simulink model "Avi_PWMSYN"  (Simulink 7.3)
settings: Solver=ode23tb  StartTime=0.0  StopTime=.25  RelTol=1e-3
libraries: powerlib x24, simulink x1
settings Model: Creator=ADMIN  LastModifiedBy=ADMIN

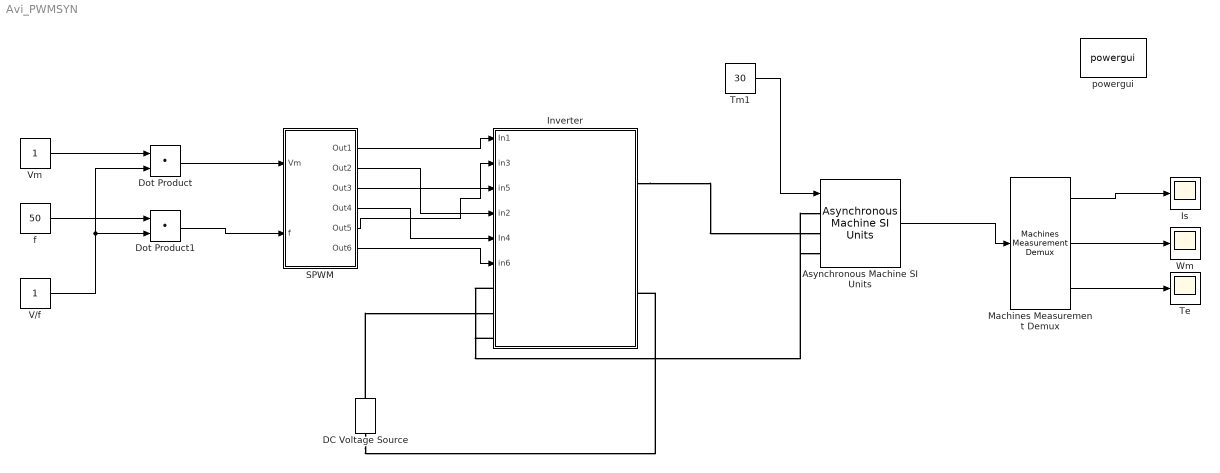
== system Avi_PWMSYN ==
  Asynchronous Machine SI Units : powerlib/Machines/Asynchronous Machine SI Units  DialogController=POWERSYS.PowerSysDialog  SystemSampleTime=-1  PresetModel=No  MechanicalLoad=Torque Tm  ShowDetailedParameters=on  RotorType=Squirrel-cage  ReferenceFrame=Stationary  NominalParameters=[ 3746 220 50 ]  Stator=[.453 2e-3]  Rotor=[ .816 2e-3]  Lm=.0631  Mechanical=[ .089 0 2 ]  PolePairs=2  InitialConditions=[1 0 0 0 0 0 0 0]  Units=SI  LoadFlowParameters=1492000  SimulateSaturation=off  Saturation=[14.03593122, 27.81365428, 53.79336849, 72.68890987, 97.98006896, 148.6815601, 215.7428561, 302.9841135, 428.7778367 ; 230, 322, 414, 460, 506, 552, 598, 644, 690]  TsPowergui=0  TsBlock=-1  IterativeModel=Forward Euler
  DC Voltage Source : powerlib/Electrical Sources/DC Voltage Source  DialogController=POWERSYS.PowerSysDialog  SystemSampleTime=-1  Amplitude=250  Measurements=None
  Dot Product : DotProduct  OutDataType=fixdt(1, 16)  OutScaling=2^-10  InputSameDT=on  OutDataTypeStr=Inherit: Inherit via internal rule
  Dot Product1 : DotProduct  OutDataType=fixdt(1, 16)  OutScaling=2^-10  InputSameDT=on  OutDataTypeStr=Inherit: Inherit via internal rule
  Inverter : Subsystem
  Is : Scope
      settings: YMin=-40  YMax=40  SaveName=ScopeData4
  Machines Measurement Demux : powerlib/Machines/Machines Measurement Demux  DialogController=POWERSYS.PowerSysDialog  SystemSampleTime=-1  machType=Asynchronous  ssm1=on  ssm2=on  ssm3=on  ssm4=on  ssm5=on  ssm6=on  sm1=on  sm2=off  sm3=off  sm4=off  sm5=off  sm6=off  sm7=off  sm8=on  sm9=off  sm10=off  sm11=off  sm115=on  sm12=off  sm13=off  sm14=off  asm1=off  asm2=off  asm3=off  asm4=off  asm5=on  asm6=off  asm7=off  asm8=off  asm9=on  asm10=on  asm11=off  pmsm1=on  pmsm2=on  pmsm3=on  pmsm4=off  pmsm5=on  pmsm6=on  pmsm7=on  lastType=1
  SPWM : Subsystem
  Te : Scope
      settings: YMin=10  YMax=100  SaveName=ScopeData6
  Tm1 : Constant  Value=30  OutDataType=fixdt(1, 16)  OutScaling=2^0
  V/f : Constant  OutDataType=fixdt(1, 16)  OutScaling=2^0
  Vm : Constant  OutDataType=fixdt(1, 16)  OutScaling=2^0
  Wm : Scope
      settings: YMin=0  YMax=20  SaveName=ScopeData5
  f : Constant  Value=50  OutDataType=fixdt(1, 16)  OutScaling=2^0
  powergui : powerlib/powergui  Priority=1  SystemSampleTime=-1  SimulationMode=Continuous  SampleTime=50e-6  frequency=60  SPID=off  DisableSnubberDevices=off  DisableRonSwitches=off  DisableVfSwitches=off  SwTol=0  Interpol=off  frequencyindice=0  echomessages=off  HookPort=off  DisplayEquations=off  FunctionMessages=off  EnableUseOfTLC=off  x0status=blocks  RestoreLinks=warning  Frange=[0:2:500]  Ylog=off  Xlog=on  ShowGrid=off  save=off  variable=ZData  ZoomFFT=on  StartTime=0.0  cycles=1  DisplayStyle=1  fundamental=60  FreqAxis=off  MaxFrequency=1000  frequencyindicesteady=1  RmsSteady=1  display=off  Ts=0  methode=off
  wires:
  Vm/1 -> Dot Product/1
  f/1 -> Dot Product1/1
  V/f/1 -> Dot Product1/2, Dot Product/2
  Dot Product/1 -> SPWM/1(Vm)
  Dot Product1/1 -> SPWM/2(f)
  SPWM/1(Out1) -> Inverter/1(In1)
  SPWM/2(Out2) -> Inverter/4(in2)
  SPWM/3(Out3) -> Inverter/2(in3)
  SPWM/4(Out4) -> Inverter/5(In4)
  SPWM/5(Out5) -> Inverter/3(in5)
  SPWM/6(Out6) -> Inverter/6(in6)
  Tm1/1 -> Asynchronous Machine SI Units/1
  Asynchronous Machine SI Units/1 -> Machines Measurement Demux/1
  Machines Measurement Demux/1 -> Is/1
  Machines Measurement Demux/2 -> Wm/1
  Machines Measurement Demux/3 -> Te/1
  connections:
  Inverter/LConn1 -- Asynchronous Machine SI Units/LConn1
  Inverter/RConn1 -- Asynchronous Machine SI Units/LConn2
  Inverter/LConn3 -- Asynchronous Machine SI Units/LConn3
  DC Voltage Source/RConn1 -- Inverter/LConn2
  DC Voltage Source/LConn1 -- Inverter/RConn2

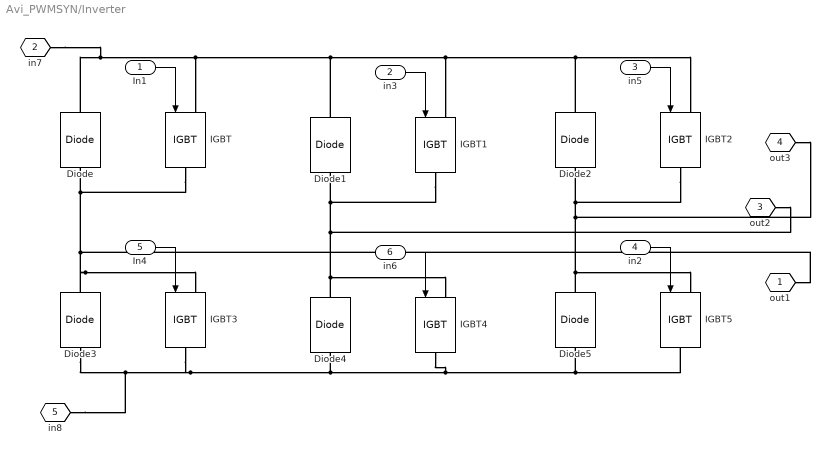
== system Avi_PWMSYN/Inverter ==
  In1 : Inport  OutDataType=fixdt(1, 16)  OutScaling=2^0
  in3 : Inport  Port=2  OutDataType=fixdt(1, 16)  OutScaling=2^0
  in5 : Inport  Port=3  OutDataType=fixdt(1, 16)  OutScaling=2^0
  in2 : Inport  Port=4  OutDataType=fixdt(1, 16)  OutScaling=2^0
  In4 : Inport  Port=5  OutDataType=fixdt(1, 16)  OutScaling=2^0
  in6 : Inport  Port=6  OutDataType=fixdt(1, 16)  OutScaling=2^0
  Diode{,1..5} (6 alike) : powerlib/Power Electronics/Diode  DialogController=POWERSYS.PowerSysDialog  SystemSampleTime=-1  Ron=0.001  Lon=0  Vf=0.8  IC=0  UseSnubber=off  Rs=500  Cs=250e-9  Measurements=off
  IGBT{,1..5} (6 alike) : powerlib/Power Electronics/IGBT  DialogController=POWERSYS.PowerSysDialog  SystemSampleTime=-1  Ron=0.001  Lon=0  Vf=1  Tf=1e-6  Tt=2e-6  IC=0  Rs=1e5  Cs=inf  Measurements=off
  out1 : PMIOPort  Tag=PMCPort  Port=1  Side=Left
  in7 : PMIOPort  Tag=PMCPort  Port=2  Side=Left
  out2 : PMIOPort  Tag=PMCPort  Port=3  Side=Right
  out3 : PMIOPort  Tag=PMCPort  Port=4  Side=Left
  in8 : PMIOPort  Tag=PMCPort  Port=5  Side=Right
  wires:
  In1/1 -> IGBT/1
  in3/1 -> IGBT1/1
  in5/1 -> IGBT2/1
  In4/1 -> IGBT3/1
  in6/1 -> IGBT4/1
  in2/1 -> IGBT5/1
  connections:
  out1/RConn1 -- Diode3/RConn1 -- IGBT3/LConn1 -- Diode/LConn1 -- IGBT/RConn1
  Diode/RConn1 -- in7/RConn1 -- IGBT1/LConn1 -- IGBT2/LConn1 -- Diode2/RConn1 -- Diode1/RConn1 -- IGBT/LConn1
  IGBT1/RConn1 -- Diode1/LConn1 -- Diode4/RConn1 -- IGBT4/LConn1 -- out2/RConn1
  IGBT2/RConn1 -- Diode2/LConn1 -- Diode5/RConn1 -- IGBT5/LConn1 -- out3/RConn1
  Diode3/LConn1 -- in8/RConn1 -- Diode5/LConn1 -- IGBT5/RConn1 -- IGBT4/RConn1 -- Diode4/LConn1 -- IGBT3/RConn1

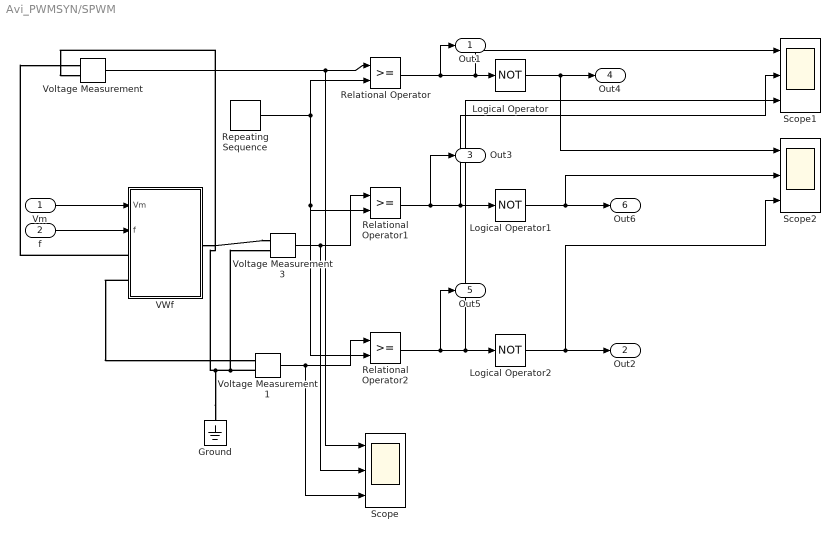
== system Avi_PWMSYN/SPWM ==
  Vm : Inport  OutDataType=fixdt(1, 16)  OutScaling=2^0
  f : Inport  Port=2  OutDataType=fixdt(1, 16)  OutScaling=2^0
  Ground : powerlib/Elements/Ground  DialogController=POWERSYS.PowerSysDialog  PhysicalDomain=powersysdomain  SubClassName=unknown  LeftPortType=p1  RightPortType=p1  LConnTagsString=a
  Logical Operator : Logic  Operator=NOT  AllPortsSameDT=off  OutDataTypeMode=boolean  LogicDataType=fixdt(0, 8)  OutDataTypeStr=boolean
  Logical Operator1 : Logic  Operator=NOT  AllPortsSameDT=off  OutDataTypeMode=boolean  LogicDataType=fixdt(0, 8)  OutDataTypeStr=boolean
  Logical Operator2 : Logic  Operator=NOT  AllPortsSameDT=off  OutDataTypeMode=boolean  LogicDataType=fixdt(0, 8)  OutDataTypeStr=boolean
  Relational Operator : RelationalOperator  LogicOutDataTypeMode=boolean  LogicDataType=fixdt(0, 8)  OutDataTypeStr=boolean
  Relational Operator1 : RelationalOperator  LogicOutDataTypeMode=boolean  LogicDataType=fixdt(0, 8)  OutDataTypeStr=boolean
  Relational Operator2 : RelationalOperator  LogicOutDataTypeMode=boolean  LogicDataType=fixdt(0, 8)  OutDataTypeStr=boolean
  Repeating Sequence : simulink/Sources/Repeating Sequence  SystemSampleTime=-1  rep_seq_t=[0 .0005 .0015 .002]  rep_seq_y=[0 1 -1 0]
  Scope : Scope  NumInputPorts=3
      settings: YMin=-5~-5~-5  YMax=5~5~5
  Scope1 : Scope  NumInputPorts=3
      settings: YMin=-5~-5~-5  YMax=5~5~5  SaveName=ScopeData2
  Scope2 : Scope  NumInputPorts=3
      settings: YMin=-5~-5~-5  YMax=5~5~5  SaveName=ScopeData3
  VWf : Subsystem
  Voltage Measurement : powerlib/Measurements/Voltage Measurement  DialogController=POWERSYS.PowerSysDialog  SystemSampleTime=-1  PhasorSimulation=off  OutputType=Complex  PSBequivalent=0
  Voltage Measurement1 : powerlib/Measurements/Voltage Measurement  DialogController=POWERSYS.PowerSysDialog  SystemSampleTime=-1  PhasorSimulation=off  OutputType=Complex  PSBequivalent=0
  Voltage Measurement3 : powerlib/Measurements/Voltage Measurement  DialogController=POWERSYS.PowerSysDialog  SystemSampleTime=-1  PhasorSimulation=off  OutputType=Complex  PSBequivalent=0
  Out1 : Outport  OutDataType=fixdt(1, 16)  OutScaling=2^0
  Out2 : Outport  Port=2  OutDataType=fixdt(1, 16)  OutScaling=2^0
  Out3 : Outport  Port=3  OutDataType=fixdt(1, 16)  OutScaling=2^0
  Out4 : Outport  Port=4  OutDataType=fixdt(1, 16)  OutScaling=2^0
  Out5 : Outport  Port=5  OutDataType=fixdt(1, 16)  OutScaling=2^0
  Out6 : Outport  Port=6  OutDataType=fixdt(1, 16)  OutScaling=2^0
  wires:
  Vm/1 -> VWf/1(Vm)
  f/1 -> VWf/2(f)
  Voltage Measurement/1 -> Relational Operator/1, Scope/1
  Repeating Sequence/1 -> Relational Operator/2, Relational Operator1/2, Relational Operator2/2
  Voltage Measurement3/1 -> Relational Operator1/1, Scope/2
  Voltage Measurement1/1 -> Relational Operator2/1, Scope/3
  Relational Operator/1 -> Out1/1, Logical Operator/1, Scope1/1
  Relational Operator1/1 -> Out3/1, Logical Operator1/1, Scope1/2
  Relational Operator2/1 -> Logical Operator2/1, Scope1/3, Out5/1
  Logical Operator/1 -> Out4/1, Scope2/1
  Logical Operator1/1 -> Out6/1, Scope2/2
  Logical Operator2/1 -> Out2/1, Scope2/3
  connections:
  Ground/LConn1 -- Voltage Measurement/LConn2 -- Voltage Measurement1/LConn2 -- Voltage Measurement3/LConn2
  VWf/LConn1 -- Voltage Measurement/LConn1
  VWf/LConn2 -- Voltage Measurement1/LConn1
  VWf/RConn1 -- Voltage Measurement3/LConn1

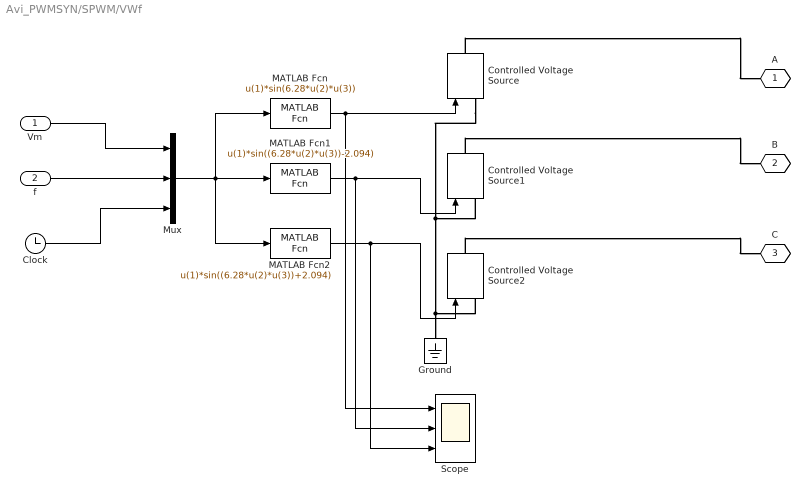
== system Avi_PWMSYN/SPWM/VWf ==
  Vm : Inport  OutDataType=fixdt(1, 16)  OutScaling=2^0
  f : Inport  Port=2  OutDataType=fixdt(1, 16)  OutScaling=2^0
  Clock : Clock
      settings: Decimation=10
  Controlled Voltage Source : powerlib/Electrical Sources/Controlled Voltage Source  DialogController=POWERSYS.PowerSysDialog  SystemSampleTime=-1  Initialize=on  Source_Type=AC  Amplitude=0  Phase=0  Frequency=0  Measurements=None
  Controlled Voltage Source1 : powerlib/Electrical Sources/Controlled Voltage Source  DialogController=POWERSYS.PowerSysDialog  SystemSampleTime=-1  Initialize=on  Source_Type=AC  Amplitude=0  Phase=0  Frequency=0  Measurements=None
  Controlled Voltage Source2 : powerlib/Electrical Sources/Controlled Voltage Source  DialogController=POWERSYS.PowerSysDialog  SystemSampleTime=-1  Initialize=on  Source_Type=AC  Amplitude=0  Phase=0  Frequency=0  Measurements=None
  Ground : powerlib/Elements/Ground  DialogController=POWERSYS.PowerSysDialog  PhysicalDomain=powersysdomain  SubClassName=unknown  LeftPortType=p1  RightPortType=p1  LConnTagsString=a
  MATLAB Fcn : MATLABFcn  MATLABFcn=u(1)*sin(6.28*u(2)*u(3))
  MATLAB Fcn1 : MATLABFcn  MATLABFcn=u(1)*sin((6.28*u(2)*u(3))-2.094)
  MATLAB Fcn2 : MATLABFcn  MATLABFcn=u(1)*sin((6.28*u(2)*u(3))+2.094)
  Mux : Mux  Inputs=3
  Scope : Scope  NumInputPorts=3
      settings: TimeRange=0.25  YMin=-5~-5~-5  YMax=5~5~5
  A : PMIOPort  Tag=PMCPort  Port=1  Side=Left
  B : PMIOPort  Tag=PMCPort  Port=2  Side=Right
  C : PMIOPort  Tag=PMCPort  Port=3  Side=Left
  wires:
  MATLAB Fcn2/1 -> Controlled Voltage Source2/1, Scope/3
  MATLAB Fcn1/1 -> Controlled Voltage Source1/1, Scope/2
  MATLAB Fcn/1 -> Controlled Voltage Source/1, Scope/1
  Mux/1 -> MATLAB Fcn/1, MATLAB Fcn1/1, MATLAB Fcn2/1
  Clock/1 -> Mux/3
  f/1 -> Mux/2
  Vm/1 -> Mux/1
  connections:
  Controlled Voltage Source/LConn1 -- Ground/LConn1 -- Controlled Voltage Source2/LConn1 -- Controlled Voltage Source1/LConn1
  Controlled Voltage Source/RConn1 -- A/RConn1
  Controlled Voltage Source1/RConn1 -- B/RConn1
  Controlled Voltage Source2/RConn1 -- C/RConn1
